simulink model "app_Main10msMgr"  (R2019b)
settings: Solver=FixedStepDiscrete  StartTime=0.0  StopTime=inf  FixedStep=0.01  RelTol=1e-3  EnableMultiTasking=on
PreLoadFcn:
  | try
  |    tapas_types('load');
  | catch
  |   disp('TAPAS WARNING: Tapas Types could not be loaded ...');
  | end
  | 
  | try
  |   app_types('load');
  | catch
  |   currdir =pwd;
  |   try
  |     cd('..\app_types\');
  |     app_types('load');
  |     cd(currdir);
  |   catch
  |     try
  |        cd('..\..\app_types\');
  |        app_types('load');
  |        cd(currdir);
  |     catch
  |        cd(currdir);
  |        disp('TAPAS WARNING: Application Types could not be loaded ...');
  |     end
  |   end
  |   try
  |       clear currdir;
  |   catch
  |      %Do nothing
  |   end
  | end
libraries: Lib_SiftProbe_deVCU_IO x44, Lib_SiftProbe_deVCU_Anlg x23, Lib_SiftProbe_deVCU_Com x4, simulink x4, hdlsllib x1
settings Model: Creator=kmansour  LastModifiedBy=depl_
settings DataIOCC: LimitDataPoints=on  SaveFormat=Array  ReturnWorkspaceOutputs=off
settings OptimizationCC: LifeSpan=1  EfficientTunableParamExpr=on
settings DebuggingCC: AllowSymbolicDim=off  SFUnexpectedBacktrackingDiag=warning  SFNoUnconditionalDefaultTransitionDiag=warning  SFExecutionAtInitializationDiag=none  ArithmeticOperatorsInVariantConditions=warning
settings HardwareCC: ProdBitPerPointer=32  ProdBitPerSizeT=32  ProdBitPerPtrDiffT=32  ProdLargestAtomicInteger=Long  ProdLargestAtomicFloat=Double  ProdEndianess=BigEndian  ProdWordSize=32  ProdHWDeviceType=Texas Instruments->TMS570 Cortex-R4
settings ModelReferenceCC: ModelReferenceNumInstancesAllowed=Single  PropagateSignalLabelsOutOfModel=off
settings SFSimCC: SimUseLocalCustomCode=off  MATLABDynamicMemAlloc=off  CustomCodeUndefinedFunction=UseInterfaceOnly
settings RTWCC: SystemTargetFile=ert.tlc  GenCodeOnly=on  TemplateMakefile=ert_default_tmf  GenerateReport=on  RTWUseLocalCustomCode=off  IncludeHyperlinkInReport=on  LaunchReport=on  GenerateTraceInfo=on  GenerateTraceReport=on  GenerateTraceReportSl=on  GenerateTraceReportSf=on  GenerateTraceReportEml=on  CheckMdlBeforeBuild=Warning
settings CodeAppCC: IgnoreCustomStorageClasses=off  MaxIdLength=63  StateflowObjectComments=on
settings ERTTargetCC: MultiwordLength=2048  GenerateSampleERTMain=on  SuppressErrorStatus=on  GenerateASAP2=on  RTWCAPISignals=on  RTWCAPIParams=on  RTWCAPIStates=on  RTWCAPIRootIO=on  ERTSrcFileBannerTemplate=deMCD_code_template.cgt  ERTHdrFileBannerTemplate=deMCD_code_template.cgt  ERTDataSrcFileTemplate=deMCD_code_template.cgt  ERTDataHdrFileTemplate=deMCD_code_template.cgt  ERTCustomFileTemplate=example_file_process.tlc  ConvertIfToSwitch=off  SuppressUnreachableDefaultCases=off
settings ConfigComp: CovMetricSettings=dw  CovHtmlReporting=on  CovSaveCumulativeToWorkspaceVar=on  CovSaveSingleToWorkspaceVar=on  CovExternalEMLEnable=off

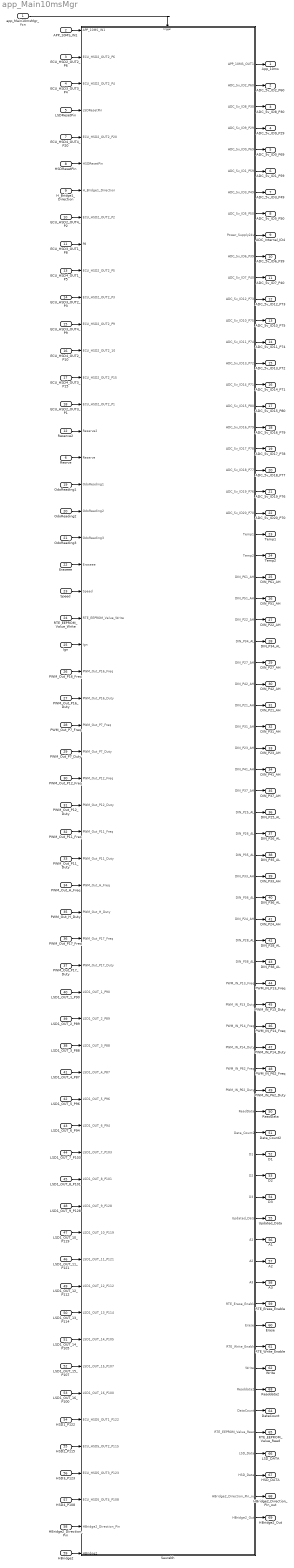
== system app_Main10msMgr ==
  app_Main10msMgr_fcn : Inport  SampleTime=10e-3  OutputFunctionCall=on
  APP_10MS_IN1 : Inport  Port=2
  ECU_HSD2_OUT2_P6 : Inport  Port=3
  ECU_HSD3_OUT3_P4 : Inport  Port=4
  LSDResetPin : Inport  Port=5
  Resrve : Inport  Port=6
  ECU_HSD4_OUT4_P20 : Inport  Port=7
  HSDResetPin : Inport  Port=8
  H_Bridge1_Direction : Inport  Port=9
  ECU_HSD2_OUT4_P2 : Inport  Port=10
  ECU_HSD3_OUT1_P8 : Inport  Port=11
  Reserve2 : Inport  Port=12
  ECU_HSD4_OUT1_P5 : Inport  Port=13
  ECU_HSD3_OUT2_P3 : Inport  Port=14
  ECU_HSD3_OUT4_P9 : Inport  Port=15
  ECU_HSD4_OUT2_P10 : Inport  Port=16
  ECU_HSD4_OUT3_P15 : Inport  Port=17
  ECU_HSD2_OUT3_P1 : Inport  Port=18
  OdoReading1 : Inport  Port=19
  OdoReading2 : Inport  Port=20
  OdoReading3 : Inport  Port=21
  Eraseee : Inport  Port=22
  Speed : Inport  Port=23
  RTE_EEPROM_Value_Write : Inport  Port=24
  Ign : Inport  Port=25
  PWM_Out_P16_Freq : Inport  Port=26
  PWM_Out_P16_Duty : Inport  Port=27
  PWM_Out_P7_Freq : Inport  Port=28
  PWM_Out_P7_Duty : Inport  Port=29
  PWM_Out_P12_Freq : Inport  Port=30
  PWM_Out_P12_Duty : Inport  Port=31
  PWM_Out_P11_Freq : Inport  Port=32
  PWM_Out_P11_Duty : Inport  Port=33
  PWM_Out_H_Freq : Inport  Port=34
  PWM_Out_H_Duty : Inport  Port=35
  PWM_Out_P17_Freq : Inport  Port=36
  PWM_Out_P17_Duty : Inport  Port=37
  LSD1_OUT_3_P88 : Inport  Port=38
  LSD1_OUT_2_P89 : Inport  Port=39
  LSD1_OUT_1_P90 : Inport  Port=40
  LSD1_OUT_4_P87 : Inport  Port=41
  LSD1_OUT_5_P96 : Inport  Port=42
  LSD1_OUT_6_P94 : Inport  Port=43
  LSD1_OUT_7_P103 : Inport  Port=44
  LSD1_OUT_8_P101 : Inport  Port=45
  LSD1_OUT_11_P121 : Inport  Port=46
  LSD1_OUT_10_P119 : Inport  Port=47
  LSD1_OUT_9_P128 : Inport  Port=48
  LSD1_OUT_12_P112 : Inport  Port=49
  LSD1_OUT_13_P114 : Inport  Port=50
  LSD1_OUT_14_P105 : Inport  Port=51
  LSD1_OUT_15_P107 : Inport  Port=52
  LSD1_OUT_16_P100 : Inport  Port=53
  HSD1_P122 : Inport  Port=54
  HSD2_P115 : Inport  Port=55
  HSD3_P123 : Inport  Port=56
  HSD4_P108 : Inport  Port=57
  HBridge2_Direction_Pin : Inport  Port=58
  HBridge2 : Inport  Port=59
  Saurabh : Subsystem
      mask Display: image(('Devise Logo.JPG'),'center');
  App_10ms : Outport
  ADC_5v_ID2_P60 : Outport  Port=2
  ADC_5v_ID8_P30 : Outport  Port=3
  ADC_5v_ID9_P29 : Outport  Port=4
  ADC_5v_ID0_P69 : Outport  Port=5
  ADC_5v_ID1_P59 : Outport  Port=6
  ADC_5v_ID3_P49 : Outport  Port=7
  ADC_5v_ID5_P50 : Outport  Port=8
  ADC_Internal_ID4 : Outport  Port=9
  ADC_5v_ID6_P39 : Outport  Port=10
  ADC_5v_ID7_P40 : Outport  Port=11
  ADC_5v_ID12_P73 : Outport  Port=12
  ADC_5v_ID10_P75 : Outport  Port=13
  ADC_5v_ID11_P74 : Outport  Port=14
  ADC_5v_ID13_P72 : Outport  Port=15
  ADC_5v_ID14_P71 : Outport  Port=16
  ADC_5v_ID15_P80 : Outport  Port=17
  ADC_5v_ID16_P79 : Outport  Port=18
  ADC_5v_ID17_P78 : Outport  Port=19
  ADC_5v_ID18_P77 : Outport  Port=20
  ADC_5v_ID19_P76 : Outport  Port=21
  ADC_5v_ID20_P70 : Outport  Port=22
  Temp1 : Outport  Port=23
  Temp2 : Outport  Port=24
  DIN_P61_AH : Outport  Port=25
  DIN_P51_AH : Outport  Port=26
  DIN_P22_AH : Outport  Port=27
  DIN_P34_AL : Outport  Port=28
  DIN_P27_AH : Outport  Port=29
  DIN_P42_AH : Outport  Port=30
  DIN_P21_AH : Outport  Port=31
  DIN_P31_AH : Outport  Port=32
  DIN_P23_AH : Outport  Port=33
  DIN_P41_AH : Outport  Port=34
  DIN_P37_AH : Outport  Port=35
  DIN_P25_AL : Outport  Port=36
  DIN_P26_AL : Outport  Port=37
  DIN_P35_AL : Outport  Port=38
  DIN_P33_AH : Outport  Port=39
  DIN_P36_AL : Outport  Port=40
  DIN_P24_AH : Outport  Port=41
  DIN_P28_AL : Outport  Port=42
  DIN_P38_AL : Outport  Port=43
  PWM_IN_P13_Freq : Outport  Port=44
  PWM_IN_P13_Duty : Outport  Port=45
  PWM_IN_P14_Freq : Outport  Port=46
  PWM_IN_P14_Duty : Outport  Port=47
  PWM_IN_P62_Freq : Outport  Port=48
  PWM_IN_P62_Duty : Outport  Port=49
  ReadData : Outport  Port=50
  Data_Count2 : Outport  Port=51
  D1 : Outport  Port=52
  D2 : Outport  Port=53
  D3 : Outport  Port=54
  Updated_Data : Outport  Port=55
  A1 : Outport  Port=56
  A2 : Outport  Port=57
  A3 : Outport  Port=58
  RTE_Erase_Enable : Outport  Port=59
  Erase : Outport  Port=60
  RTE_Write_Enable : Outport  Port=61
  Write : Outport  Port=62
  Readdata2 : Outport  Port=63
  DataCount : Outport  Port=64
  RTE_EEPROM_Value_Read : Outport  Port=65
  LSD_DATA : Outport  Port=66
  HSD_DATA : Outport  Port=67
  HBridge2_Direction_Pin_out : Outport  Port=68
  HBridge2_Out : Outport  Port=69
  wires:
  Saurabh/44(PWM_IN_P13_Freq) -> PWM_IN_P13_Freq/1
  Saurabh/67(HSD_Data) -> HSD_DATA/1
  Saurabh/62(Write) -> Write/1
  Saurabh/66(LSD_Data) -> LSD_DATA/1
  LSD1_OUT_13_P114/1 -> Saurabh/49("LSD1_OUT_13_P114 ")
  LSD1_OUT_1_P90/1 -> Saurabh/37(LSD1_OUT_1_P90)
  LSD1_OUT_12_P112/1 -> Saurabh/48("LSD1_OUT_12_P112 ")
  Eraseee/1 -> Saurabh/21(Eraseee)
  Saurabh/53(D2) -> D2/1
  OdoReading1/1 -> Saurabh/18(OdoReading1)
  Saurabh/40(DIN_P36_AL) -> DIN_P36_AL/1
  PWM_Out_P17_Freq/1 -> Saurabh/35(PWM_Out_P17_Freq)
  LSD1_OUT_10_P119/1 -> Saurabh/46("LSD1_OUT_10_P119 ")
  LSD1_OUT_9_P128/1 -> Saurabh/45("LSD1_OUT_9_P128 ")
  LSD1_OUT_8_P101/1 -> Saurabh/44("LSD1_OUT_8_P101 ")
  LSD1_OUT_14_P105/1 -> Saurabh/50("LSD1_OUT_14_P105 ")
  PWM_Out_H_Freq/1 -> Saurabh/33(PWM_Out_H_Freq)
  LSD1_OUT_15_P107/1 -> Saurabh/51("LSD1_OUT_15_P107 ")
  LSD1_OUT_11_P121/1 -> Saurabh/47("LSD1_OUT_11_P121 ")
  Ign/1 -> Saurabh/24(Ign)
  PWM_Out_P11_Freq/1 -> Saurabh/31(PWM_Out_P11_Freq)
  LSD1_OUT_16_P100/1 -> Saurabh/52(LSD1_OUT_16_P100)
  LSD1_OUT_6_P94/1 -> Saurabh/42("LSD1_OUT_6_P94 ")
  PWM_Out_P16_Freq/1 -> Saurabh/25(PWM_Out_P16_Freq)
  LSD1_OUT_2_P89/1 -> Saurabh/38(LSD1_OUT_2_P89)
  PWM_Out_P7_Duty/1 -> Saurabh/28(PWM_Out_P7_Duty)
  LSD1_OUT_4_P87/1 -> Saurabh/40("LSD1_OUT_4_P87 ")
  LSD1_OUT_5_P96/1 -> Saurabh/41("LSD1_OUT_5_P96 ")
  LSD1_OUT_7_P103/1 -> Saurabh/43("LSD1_OUT_7_P103 ")
  LSD1_OUT_3_P88/1 -> Saurabh/39("LSD1_OUT_3_P88 ")
  PWM_Out_P12_Freq/1 -> Saurabh/29(PWM_Out_P12_Freq)
  PWM_Out_P16_Duty/1 -> Saurabh/26(PWM_Out_P16_Duty)
  PWM_Out_P7_Freq/1 -> Saurabh/27(PWM_Out_P7_Freq)
  PWM_Out_P17_Duty/1 -> Saurabh/36(PWM_Out_P17_Duty)
  PWM_Out_H_Duty/1 -> Saurabh/34(PWM_Out_H_Duty)
  PWM_Out_P11_Duty/1 -> Saurabh/32(PWM_Out_P11_Duty)
  PWM_Out_P12_Duty/1 -> Saurabh/30(PWM_Out_P12_Duty)
  Saurabh/65(RTE_EEPROM_Value_Read) -> RTE_EEPROM_Value_Read/1
  Saurabh/64(DataCount) -> DataCount/1
  Speed/1 -> Saurabh/22(Speed)
  Saurabh/63(Readdata2) -> Readdata2/1
  Saurabh/61(RTE_Write_Enable) -> RTE_Write_Enable/1
  RTE_EEPROM_Value_Write/1 -> Saurabh/23(RTE_EEPROM_Value_Write)
  ECU_HSD4_OUT4_P20/1 -> Saurabh/5(ECU_HSD2_OUT2_P20)
  Saurabh/60(Erase) -> Erase/1
  Saurabh/59(RTE_Erase_Enable) -> RTE_Erase_Enable/1
  Saurabh/55(Updated_Data) -> Updated_Data/1
  Saurabh/58(A3) -> A3/1
  Saurabh/48(PWM_IN_P62_Freq) -> PWM_IN_P62_Freq/1
  Saurabh/57(A2) -> A2/1
  Saurabh/56(A1) -> A1/1
  Saurabh/52(D1) -> D1/1
  Saurabh/54(D3) -> D3/1
  Saurabh/46(PWM_IN_P14_Freq) -> PWM_IN_P14_Freq/1
  Saurabh/51(Data_Count2) -> Data_Count2/1
  Saurabh/50(ReadData) -> ReadData/1
  OdoReading2/1 -> Saurabh/19(OdoReading2)
  OdoReading3/1 -> Saurabh/20(OdoReading3)
  Saurabh/47(PWM_IN_P14_Duty) -> PWM_IN_P14_Duty/1
  Saurabh/49(PWM_IN_P62_Duty) -> PWM_IN_P62_Duty/1
  Saurabh/45(PWM_IN_P13_Duty) -> PWM_IN_P13_Duty/1
  Saurabh/36(DIN_P25_AL) -> DIN_P25_AL/1
  Saurabh/39(DIN_P33_AH) -> DIN_P33_AH/1
  Saurabh/42(DIN_P28_AL) -> DIN_P28_AL/1
  Saurabh/38(DIN_P35_AL) -> DIN_P35_AL/1
  Saurabh/37(DIN_P26_AL) -> DIN_P26_AL/1
  Saurabh/41(DIN_P24_AH) -> DIN_P24_AH/1
  Saurabh/35(DIN_P37_AH) -> DIN_P37_AH/1
  Saurabh/43(DIN_P38_AL) -> DIN_P38_AL/1
  Saurabh/29(DIN_P27_AH) -> DIN_P27_AH/1
  Saurabh/25(DIN_P61_AH) -> DIN_P61_AH/1
  Saurabh/31(DIN_P21_AH) -> DIN_P21_AH/1
  Saurabh/34(DIN_P41_AH) -> DIN_P41_AH/1
  Saurabh/32(DIN_P31_AH) -> DIN_P31_AH/1
  Saurabh/26(DIN_P51_AH) -> DIN_P51_AH/1
  Saurabh/30(DIN_P42_AH) -> DIN_P42_AH/1
  Saurabh/27(DIN_P22_AH) -> DIN_P22_AH/1
  Saurabh/28(DIN_P34_AL) -> DIN_P34_AL/1
  Saurabh/33(DIN_P23_AH) -> DIN_P23_AH/1
  ECU_HSD2_OUT3_P1/1 -> Saurabh/15(ECU_HSD2_OUT2_P1)
  ECU_HSD4_OUT2_P10/1 -> Saurabh/13(ECU_HSD2_OUT2_10)
  ECU_HSD4_OUT1_P5/1 -> Saurabh/10(ECU_HSD2_OUT2_P5)
  ECU_HSD3_OUT4_P9/1 -> Saurabh/12(ECU_HSD2_OUT2_P9)
  ECU_HSD3_OUT2_P3/1 -> Saurabh/11(ECU_HSD2_OUT2_P3)
  ECU_HSD4_OUT3_P15/1 -> Saurabh/14(ECU_HSD2_OUT2_P15)
  Reserve2/1 -> Saurabh/16(Reserve2)
  ECU_HSD3_OUT1_P8/1 -> Saurabh/9(P8)
  ECU_HSD2_OUT4_P2/1 -> Saurabh/8(ECU_HSD2_OUT2_P2)
  H_Bridge1_Direction/1 -> Saurabh/7(H_Bridge1_Direction)
  HSDResetPin/1 -> Saurabh/6(HSDResetPin)
  Resrve/1 -> Saurabh/17(Reserve)
  LSDResetPin/1 -> Saurabh/4(LSDResetPin)
  ECU_HSD3_OUT3_P4/1 -> Saurabh/3(ECU_HSD2_OUT2_P4)
  ECU_HSD2_OUT2_P6/1 -> Saurabh/2(ECU_HSD2_OUT2_P6)
  Saurabh/24(Temp2) -> Temp2/1
  Saurabh/23(Temp1) -> Temp1/1
  Saurabh/15(ADC_5v_ID13_P72) -> ADC_5v_ID13_P72/1
  Saurabh/18(ADC_5v_ID16_P79) -> ADC_5v_ID16_P79/1
  Saurabh/14(ADC_5v_ID11_P74) -> ADC_5v_ID11_P74/1
  Saurabh/16(ADC_5v_ID14_P71) -> ADC_5v_ID14_P71/1
  Saurabh/22(ADC_5v_ID20_P70) -> ADC_5v_ID20_P70/1
  Saurabh/21(ADC_5v_ID19_P76) -> ADC_5v_ID19_P76/1
  Saurabh/20(ADC_5v_ID18_P77) -> ADC_5v_ID18_P77/1
  Saurabh/17(ADC_5v_ID15_P80) -> ADC_5v_ID15_P80/1
  Saurabh/19(ADC_5v_ID17_P78) -> ADC_5v_ID17_P78/1
  Saurabh/12(ADC_5v_ID12_P73) -> ADC_5v_ID12_P73/1
  Saurabh/10(ADC_5v_ID6_P39) -> ADC_5v_ID6_P39/1
  Saurabh/6(ADC_5v_ID1_P59) -> ADC_5v_ID1_P59/1
  Saurabh/13(ADC_5v_ID10_P75) -> ADC_5v_ID10_P75/1
  Saurabh/9(Power_Supply24v) -> ADC_Internal_ID4/1
  Saurabh/2(ADC_5v_ID2_P60) -> ADC_5v_ID2_P60/1
  Saurabh/11(ADC_5v_ID7_P40) -> ADC_5v_ID7_P40/1
  Saurabh/7(ADC_5v_ID3_P49) -> ADC_5v_ID3_P49/1
  Saurabh/8(ADC_5v_ID5_P50) -> ADC_5v_ID5_P50/1
  Saurabh/4(ADC_5v_ID9_P29) -> ADC_5v_ID9_P29/1
  Saurabh/3(ADC_5v_ID8_P30) -> ADC_5v_ID8_P30/1
  Saurabh/5(ADC_5v_ID0_P69) -> ADC_5v_ID0_P69/1
  Saurabh/1(APP_10MS_OUT1) -> App_10ms/1
  APP_10MS_IN1/1 -> Saurabh/1(APP_10MS_IN1)
  app_Main10msMgr_fcn/1 -> Saurabh/Trigger
  HSD1_P122/1 -> Saurabh/53(ECU_HSD5_OUT1_P122)
  HSD2_P115/1 -> Saurabh/54(ECU_HSD5_OUT2_P115)
  HSD3_P123/1 -> Saurabh/55("ECU_HSD5_OUT3_P123 ")
  HSD4_P108/1 -> Saurabh/56(ECU_HSD5_OUT4_P108)
  HBridge2_Direction_Pin/1 -> Saurabh/57(HBridge2_Direction_Pin)
  HBridge2/1 -> Saurabh/58(HBridge2)
  Saurabh/68(HBridge2_Direction_Pin_out) -> HBridge2_Direction_Pin_out/1
  Saurabh/69(HBridge2_Out) -> HBridge2_Out/1

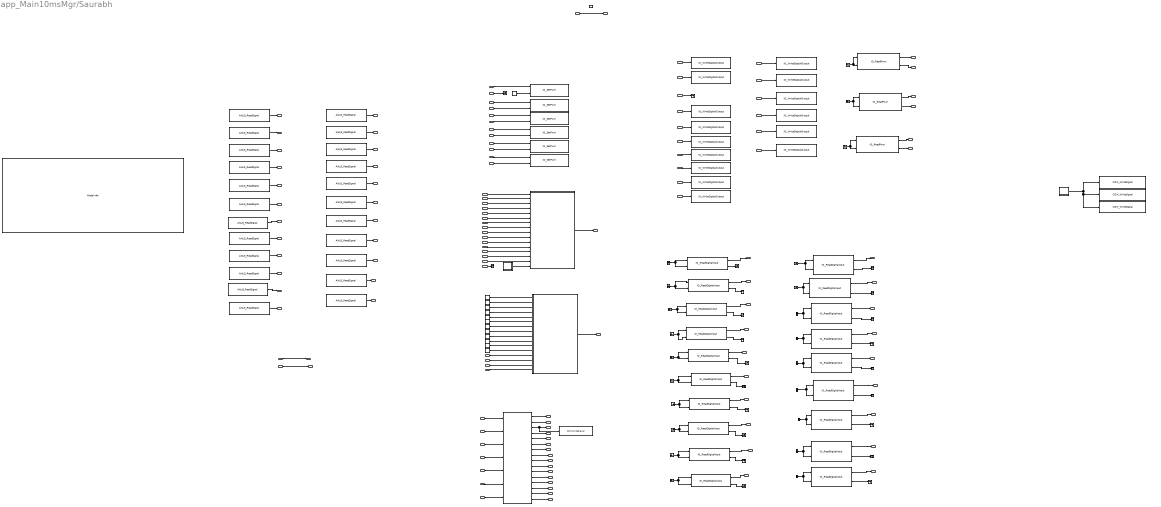
== system app_Main10msMgr/Saurabh ==
  note: CAN_Channel
  note: H_bridge2
  note: HSD
  note: LSD
  note: PWM_IN
  note: EPROM
  note: DigitalInputs
  note: DigitalOutput
  note: PWMOut
  note: ADC
  note: (C) 2020-2021 Devise Electronics Pvt Ltd
      | All rights reserved.
      |
      | All data and information contained in or disclosed by this document is confidential and proprietary information of Devise Electronics Pvt Ltd and all rights therein are expressly reserved. By accepting this material the recipient agrees that this material and the information contained therein is held in confidence and in trust and will not be used, copied, reproduced in whole or in part, nor its contents revealed in any manner to others without the express written permission of Devise Electronics Pvt Ltd
      |
      | Author:
      |
      | Devise Electronics Pvt Ltd
      | Pune,
      | India
      | E-mail: Shekhar.malani@deviseelectronics.com
  APP_10MS_IN1 : Inport
  ECU_HSD2_OUT2_P6 : Inport  Port=2
  ECU_HSD2_OUT2_P4 : Inport  Port=3
  LSDResetPin : Inport  Port=4
  ECU_HSD2_OUT2_P20 : Inport  Port=5
  HSDResetPin : Inport  Port=6
  H_Bridge1_Direction : Inport  Port=7
  ECU_HSD2_OUT2_P2 : Inport  Port=8
  P8 : Inport  Port=9
  ECU_HSD2_OUT2_P5 : Inport  Port=10
  ECU_HSD2_OUT2_P3 : Inport  Port=11
  ECU_HSD2_OUT2_P9 : Inport  Port=12
  ECU_HSD2_OUT2_10 : Inport  Port=13
  ECU_HSD2_OUT2_P15 : Inport  Port=14
  ECU_HSD2_OUT2_P1 : Inport  Port=15
  Reserve2 : Inport  Port=16
  Reserve : Inport  Port=17
  OdoReading1 : Inport  Port=18
  OdoReading2 : Inport  Port=19
  OdoReading3 : Inport  Port=20
  Eraseee : Inport  Port=21
  Speed : Inport  Port=22
  RTE_EEPROM_Value_Write : Inport  Port=23
  Ign : Inport  Port=24
  PWM_Out_P16_Freq : Inport  Port=25
  PWM_Out_P16_Duty : Inport  Port=26
  PWM_Out_P7_Freq : Inport  Port=27
  PWM_Out_P7_Duty : Inport  Port=28
  PWM_Out_P12_Freq : Inport  Port=29
  PWM_Out_P12_Duty : Inport  Port=30
  PWM_Out_P11_Freq : Inport  Port=31
  PWM_Out_P11_Duty : Inport  Port=32
  PWM_Out_H_Freq : Inport  Port=33
  PWM_Out_H_Duty : Inport  Port=34
  PWM_Out_P17_Freq : Inport  Port=35
  PWM_Out_P17_Duty : Inport  Port=36
  LSD1_OUT_1_P90 : Inport  Port=37
  LSD1_OUT_2_P89 : Inport  Port=38
  "LSD1_OUT_3_P88 " : Inport  Port=39
  "LSD1_OUT_4_P87 " : Inport  Port=40
  "LSD1_OUT_5_P96 " : Inport  Port=41
  "LSD1_OUT_6_P94 " : Inport  Port=42
  "LSD1_OUT_7_P103 " : Inport  Port=43
  "LSD1_OUT_8_P101 " : Inport  Port=44
  "LSD1_OUT_9_P128 " : Inport  Port=45
  "LSD1_OUT_10_P119 " : Inport  Port=46
  "LSD1_OUT_11_P121 " : Inport  Port=47
  "LSD1_OUT_12_P112 " : Inport  Port=48
  "LSD1_OUT_13_P114 " : Inport  Port=49
  "LSD1_OUT_14_P105 " : Inport  Port=50
  "LSD1_OUT_15_P107 " : Inport  Port=51
  LSD1_OUT_16_P100 : Inport  Port=52
  ECU_HSD5_OUT1_P122 : Inport  Port=53
  ECU_HSD5_OUT2_P115 : Inport  Port=54
  "ECU_HSD5_OUT3_P123 " : Inport  Port=55
  ECU_HSD5_OUT4_P108 : Inport  Port=56
  HBridge2_Direction_Pin : Inport  Port=57
  HBridge2 : Inport  Port=58
  Trigger : TriggerPort  TriggerType=function-call  VariantControl=Variant  SampleTimeType=periodic  SampleTime=-1  PortDimensions=1
  ANLG_ReadSignal : Lib_SiftProbe_deVCU_Anlg/ANLG_ReadSignal  PARAM_ID=ECU_ANLG_ADC_5V_P60
      settings: SourceProductName=deMCD - SiftProbe_deVCU
  ANLG_ReadSignal1 : Lib_SiftProbe_deVCU_Anlg/ANLG_ReadSignal  PARAM_ID=ECU_ANLG_ADC_5V_P30
      settings: SourceProductName=deMCD - SiftProbe_deVCU
  ANLG_ReadSignal10 : Lib_SiftProbe_deVCU_Anlg/ANLG_ReadSignal  PARAM_ID=ECU_ANLG_ADC_5V_P73
      settings: SourceProductName=deMCD - SiftProbe_deVCU
  ANLG_ReadSignal11 : Lib_SiftProbe_deVCU_Anlg/ANLG_ReadSignal  PARAM_ID=ECU_ANLG_ADC_5V_P75
      settings: SourceProductName=deMCD - SiftProbe_deVCU
  ANLG_ReadSignal12 : Lib_SiftProbe_deVCU_Anlg/ANLG_ReadSignal  PARAM_ID=ECU_ANLG_ADC_5V_P74
      settings: SourceProductName=deMCD - SiftProbe_deVCU
  ANLG_ReadSignal13 : Lib_SiftProbe_deVCU_Anlg/ANLG_ReadSignal  PARAM_ID=ECU_ANLG_ADC_5V_P72
      settings: SourceProductName=deMCD - SiftProbe_deVCU
  ANLG_ReadSignal14 : Lib_SiftProbe_deVCU_Anlg/ANLG_ReadSignal  PARAM_ID=ECU_ANLG_ADC_5V_P71
      settings: SourceProductName=deMCD - SiftProbe_deVCU
  ANLG_ReadSignal15 : Lib_SiftProbe_deVCU_Anlg/ANLG_ReadSignal  PARAM_ID=ECU_ANLG_ADC_5V_P80
      settings: SourceProductName=deMCD - SiftProbe_deVCU
  ANLG_ReadSignal16 : Lib_SiftProbe_deVCU_Anlg/ANLG_ReadSignal  PARAM_ID=ECU_ANLG_ADC_5V_P79
      settings: SourceProductName=deMCD - SiftProbe_deVCU
  ANLG_ReadSignal17 : Lib_SiftProbe_deVCU_Anlg/ANLG_ReadSignal  PARAM_ID=ECU_ANLG_ADC_5V_P78
      settings: SourceProductName=deMCD - SiftProbe_deVCU
  ANLG_ReadSignal18 : Lib_SiftProbe_deVCU_Anlg/ANLG_ReadSignal  PARAM_ID=ECU_ANLG_ADC_5V_P77
      settings: SourceProductName=deMCD - SiftProbe_deVCU
  ANLG_ReadSignal19 : Lib_SiftProbe_deVCU_Anlg/ANLG_ReadSignal  PARAM_ID=ECU_ANLG_ADC_5V_P76
      settings: SourceProductName=deMCD - SiftProbe_deVCU
  ANLG_ReadSignal2 : Lib_SiftProbe_deVCU_Anlg/ANLG_ReadSignal  PARAM_ID=ECU_ANLG_ADC_5V_P29
      settings: SourceProductName=deMCD - SiftProbe_deVCU
  ANLG_ReadSignal20 : Lib_SiftProbe_deVCU_Anlg/ANLG_ReadSignal  PARAM_ID=ECU_ANLG_ADC_5V_P70
      settings: SourceProductName=deMCD - SiftProbe_deVCU
  ANLG_ReadSignal21 : Lib_SiftProbe_deVCU_Anlg/ANLG_ReadSignal  PARAM_ID=ECU_ANLG_TEMP_SENSOR1
      settings: SourceProductName=deMCD - SiftProbe_deVCU
  ANLG_ReadSignal22 : Lib_SiftProbe_deVCU_Anlg/ANLG_ReadSignal  PARAM_ID=ECU_ANLG_TEMP_SENSOR2
      settings: SourceProductName=deMCD - SiftProbe_deVCU
  ANLG_ReadSignal3 : Lib_SiftProbe_deVCU_Anlg/ANLG_ReadSignal  PARAM_ID=ECU_ANLG_ADC_5V_P69
      settings: SourceProductName=deMCD - SiftProbe_deVCU
  ANLG_ReadSignal4 : Lib_SiftProbe_deVCU_Anlg/ANLG_ReadSignal  PARAM_ID=ECU_ANLG_ADC_5V_P59
      settings: SourceProductName=deMCD - SiftProbe_deVCU
  ANLG_ReadSignal5 : Lib_SiftProbe_deVCU_Anlg/ANLG_ReadSignal  PARAM_ID=ECU_ANLG_ADC_5V_P49
      settings: SourceProductName=deMCD - SiftProbe_deVCU
  ANLG_ReadSignal6 : Lib_SiftProbe_deVCU_Anlg/ANLG_ReadSignal  PARAM_ID=ECU_ANLG_ADC_5V_P50
      settings: SourceProductName=deMCD - SiftProbe_deVCU
  ANLG_ReadSignal7 : Lib_SiftProbe_deVCU_Anlg/ANLG_ReadSignal  PARAM_ID=ECU_ANLG_POWER_SUPPLY24V
      settings: SourceProductName=deMCD - SiftProbe_deVCU
  ANLG_ReadSignal8 : Lib_SiftProbe_deVCU_Anlg/ANLG_ReadSignal  PARAM_ID=ECU_ANLG_ADC_5V_P39
      settings: SourceProductName=deMCD - SiftProbe_deVCU
  ANLG_ReadSignal9 : Lib_SiftProbe_deVCU_Anlg/ANLG_ReadSignal  PARAM_ID=ECU_ANLG_ADC_5V_P40
      settings: SourceProductName=deMCD - SiftProbe_deVCU
  COM_WriteSignal49 : Lib_SiftProbe_deVCU_Com/COM_WriteSignal  PARAM_ID=APP_TX_CAN2_SIGNAL
      settings: SourceProductName=deMCD - SiftProbe_deVCU
  COM_WriteSignal50 : Lib_SiftProbe_deVCU_Com/COM_WriteSignal  PARAM_ID=APP_TX_CAN3_SIGNAL
      settings: SourceProductName=deMCD - SiftProbe_deVCU
  COM_WriteSignal52 : Lib_SiftProbe_deVCU_Com/COM_WriteSignal  PARAM_ID=APP_TX_CAN1_SIGNAL
      settings: SourceProductName=deMCD - SiftProbe_deVCU
  COM_WriteSignal53 : Lib_SiftProbe_deVCU_Com/COM_WriteSignal  PARAM_ID=APP_TX_ADC_P29
      settings: SourceProductName=deMCD - SiftProbe_deVCU
  Chart : Stateflow chart  BlockKeywords=__PRM__SERIALIZED__DATA__:Stateflow Chart,Stateflow Diagram  TreatAsAtomicUnit=on
  Chart1 : Stateflow chart  BlockKeywords=__PRM__SERIALIZED__DATA__:Stateflow Chart,Stateflow Diagram  TreatAsAtomicUnit=on
  Constant : Constant
  Constant1 : Constant
  Constant{3..11} (9 alike) : Constant  Value=0
  Constant12 : Constant  Value=50
  Constant2 : Constant
  Ground{,1..21} (22 alike) : Ground
  HSD : Subsystem
  IO_ReadDigitalInput : Lib_SiftProbe_deVCU_IO/IO_ReadDigitalInput  PARAM_ID=ECU_DIN_AUX_61_H_DI
      settings: SourceProductName=deMCD - SiftProbe_deVCU
  IO_ReadDigitalInput1 : Lib_SiftProbe_deVCU_IO/IO_ReadDigitalInput  PARAM_ID=ECU_DIN_AUX_51_H_DI
      settings: SourceProductName=deMCD - SiftProbe_deVCU
  IO_ReadDigitalInput10 : Lib_SiftProbe_deVCU_IO/IO_ReadDigitalInput  PARAM_ID=ECU_DIN_AUX_26_L_DI
      settings: SourceProductName=deMCD - SiftProbe_deVCU
  IO_ReadDigitalInput11 : Lib_SiftProbe_deVCU_IO/IO_ReadDigitalInput  PARAM_ID=ECU_DIN_AUX_35_L_DI
      settings: SourceProductName=deMCD - SiftProbe_deVCU
  IO_ReadDigitalInput12 : Lib_SiftProbe_deVCU_IO/IO_ReadDigitalInput  PARAM_ID=ECU_DIN_AUX_33_H_DI
      settings: SourceProductName=deMCD - SiftProbe_deVCU
  IO_ReadDigitalInput13 : Lib_SiftProbe_deVCU_IO/IO_ReadDigitalInput  PARAM_ID=ECU_DIN_AUX_36_L_DI
      settings: SourceProductName=deMCD - SiftProbe_deVCU
  IO_ReadDigitalInput14 : Lib_SiftProbe_deVCU_IO/IO_ReadDigitalInput  PARAM_ID=ECU_DIN_AUX_24_H_DI
      settings: SourceProductName=deMCD - SiftProbe_deVCU
  IO_ReadDigitalInput15 : Lib_SiftProbe_deVCU_IO/IO_ReadDigitalInput  PARAM_ID=ECU_DIN_AUX_23_H_DI
      settings: SourceProductName=deMCD - SiftProbe_deVCU
  IO_ReadDigitalInput16 : Lib_SiftProbe_deVCU_IO/IO_ReadDigitalInput  PARAM_ID=ECU_DIN_AUX_28_L_DI
      settings: SourceProductName=deMCD - SiftProbe_deVCU
  IO_ReadDigitalInput17 : Lib_SiftProbe_deVCU_IO/IO_ReadDigitalInput  PARAM_ID=ECU_DIN_AUX_41_H_DI
      settings: SourceProductName=deMCD - SiftProbe_deVCU
  IO_ReadDigitalInput18 : Lib_SiftProbe_deVCU_IO/IO_ReadDigitalInput  PARAM_ID=ECU_DIN_AUX_38_L_DI
      settings: SourceProductName=deMCD - SiftProbe_deVCU
  IO_ReadDigitalInput2 : Lib_SiftProbe_deVCU_IO/IO_ReadDigitalInput  PARAM_ID=ECU_DIN_AUX_22_H_DI
      settings: SourceProductName=deMCD - SiftProbe_deVCU
  IO_ReadDigitalInput3 : Lib_SiftProbe_deVCU_IO/IO_ReadDigitalInput  PARAM_ID=ECU_DIN_AUX_34_L_DI
      settings: SourceProductName=deMCD - SiftProbe_deVCU
  IO_ReadDigitalInput4 : Lib_SiftProbe_deVCU_IO/IO_ReadDigitalInput  PARAM_ID=ECU_DIN_AUX_27_H_DI
      settings: SourceProductName=deMCD - SiftProbe_deVCU
  IO_ReadDigitalInput5 : Lib_SiftProbe_deVCU_IO/IO_ReadDigitalInput  PARAM_ID=ECU_DIN_AUX_42_H_DI
      settings: SourceProductName=deMCD - SiftProbe_deVCU
  IO_ReadDigitalInput6 : Lib_SiftProbe_deVCU_IO/IO_ReadDigitalInput  PARAM_ID=ECU_DIN_AUX_21_H_DI
      settings: SourceProductName=deMCD - SiftProbe_deVCU
  IO_ReadDigitalInput7 : Lib_SiftProbe_deVCU_IO/IO_ReadDigitalInput  PARAM_ID=ECU_DIN_AUX_31_H_DI
      settings: SourceProductName=deMCD - SiftProbe_deVCU
  IO_ReadDigitalInput8 : Lib_SiftProbe_deVCU_IO/IO_ReadDigitalInput  PARAM_ID=ECU_DIN_AUX_37_H_DI
      settings: SourceProductName=deMCD - SiftProbe_deVCU
  IO_ReadDigitalInput9 : Lib_SiftProbe_deVCU_IO/IO_ReadDigitalInput  PARAM_ID=ECU_DIN_AUX_25_L_DI
      settings: SourceProductName=deMCD - SiftProbe_deVCU
  IO_ReadPwm : Lib_SiftProbe_deVCU_IO/IO_ReadPwm  PARAM_ID=ECU_PIN_NONAME_PIN_P13
      settings: SourceProductName=deMCD - SiftProbe_deVCU
  IO_ReadPwm1 : Lib_SiftProbe_deVCU_IO/IO_ReadPwm  PARAM_ID=ECU_PIN_NONAME_PIN_P14
      settings: SourceProductName=deMCD - SiftProbe_deVCU
  IO_ReadPwm2 : Lib_SiftProbe_deVCU_IO/IO_ReadPwm  PARAM_ID=ECU_PIN_NONAME_PIN_P62
      settings: SourceProductName=deMCD - SiftProbe_deVCU
  IO_SetPwm1 : Lib_SiftProbe_deVCU_IO/IO_SetPwm  PARAM_ID=ECU_POUT_PWM_POUT_P12
      settings: SourceProductName=deMCD - SiftProbe_deVCU
  IO_SetPwm2 : Lib_SiftProbe_deVCU_IO/IO_SetPwm  PARAM_ID=ECU_POUT_PWM_POUT_P11
      settings: SourceProductName=deMCD - SiftProbe_deVCU
  IO_SetPwm3 : Lib_SiftProbe_deVCU_IO/IO_SetPwm  PARAM_ID=ECU_POUT_PWM_POUT_H
      settings: SourceProductName=deMCD - SiftProbe_deVCU
  IO_SetPwm4 : Lib_SiftProbe_deVCU_IO/IO_SetPwm  PARAM_ID=ECU_POUT_PWM_POUT_P17
      settings: SourceProductName=deMCD - SiftProbe_deVCU
  IO_SetPwm5 : Lib_SiftProbe_deVCU_IO/IO_SetPwm  PARAM_ID=ECU_POUT_PWM_POUT_P16
      settings: SourceProductName=deMCD - SiftProbe_deVCU
  IO_SetPwm6 : Lib_SiftProbe_deVCU_IO/IO_SetPwm  PARAM_ID=ECU_POUT_PWM_POUT_P7
      settings: SourceProductName=deMCD - SiftProbe_deVCU
  IO_WriteDigitalOutput1 : Lib_SiftProbe_deVCU_IO/IO_WriteDigitalOutput  PARAM_ID=ECU_DOUT_ECU_HSD3_OUT3_P4
      settings: SourceProductName=deMCD - SiftProbe_deVCU
  IO_WriteDigitalOutput10 : Lib_SiftProbe_deVCU_IO/IO_WriteDigitalOutput  PARAM_ID=ECU_DOUT_ECU_HSD4_OUT1_P5
      settings: SourceProductName=deMCD - SiftProbe_deVCU
  IO_WriteDigitalOutput11 : Lib_SiftProbe_deVCU_IO/IO_WriteDigitalOutput  PARAM_ID=ECU_DOUT_ECU_HSD3_OUT2_P3
      settings: SourceProductName=deMCD - SiftProbe_deVCU
  IO_WriteDigitalOutput12 : Lib_SiftProbe_deVCU_IO/IO_WriteDigitalOutput  PARAM_ID=ECU_DOUT_ECU_HSD3_OUT4_P9
      settings: SourceProductName=deMCD - SiftProbe_deVCU
  IO_WriteDigitalOutput13 : Lib_SiftProbe_deVCU_IO/IO_WriteDigitalOutput  PARAM_ID=ECU_DOUT_ECU_HSD4_OUT2_P10
      settings: SourceProductName=deMCD - SiftProbe_deVCU
  IO_WriteDigitalOutput14 : Lib_SiftProbe_deVCU_IO/IO_WriteDigitalOutput  PARAM_ID=ECU_DOUT_ECU_HSD4_OUT3_P15
      settings: SourceProductName=deMCD - SiftProbe_deVCU
  IO_WriteDigitalOutput15 : Lib_SiftProbe_deVCU_IO/IO_WriteDigitalOutput  PARAM_ID=ECU_DOUT_ECU_HSD2_OUT3_P1
      settings: SourceProductName=deMCD - SiftProbe_deVCU
  IO_WriteDigitalOutput16 : Lib_SiftProbe_deVCU_IO/IO_WriteDigitalOutput  PARAM_ID=ECU_DOUT_ECU_HSD2_OUT2_P6
      settings: SourceProductName=deMCD - SiftProbe_deVCU
  IO_WriteDigitalOutput3 : Lib_SiftProbe_deVCU_IO/IO_WriteDigitalOutput  PARAM_ID=ECU_DOUT_NONAME_PIN_RESERVE1_
      settings: SourceProductName=deMCD - SiftProbe_deVCU
  IO_WriteDigitalOutput4 : Lib_SiftProbe_deVCU_IO/IO_WriteDigitalOutput  PARAM_ID=ECU_DOUT_NONAME_PIN_RESERVE2_
      settings: SourceProductName=deMCD - SiftProbe_deVCU
  IO_WriteDigitalOutput5 : Lib_SiftProbe_deVCU_IO/IO_WriteDigitalOutput  PARAM_ID=ECU_DOUT_ECU_HSD4_OUT4_P20
      settings: SourceProductName=deMCD - SiftProbe_deVCU
  IO_WriteDigitalOutput6 : Lib_SiftProbe_deVCU_IO/IO_WriteDigitalOutput  PARAM_ID=ECU_DOUT_HSD_RESET_PIN
      settings: SourceProductName=deMCD - SiftProbe_deVCU
  IO_WriteDigitalOutput7 : Lib_SiftProbe_deVCU_IO/IO_WriteDigitalOutput  PARAM_ID=ECU_DOUT_H_BRIDGE1_DIRECTION
      settings: SourceProductName=deMCD - SiftProbe_deVCU
  IO_WriteDigitalOutput8 : Lib_SiftProbe_deVCU_IO/IO_WriteDigitalOutput  PARAM_ID=ECU_DOUT_ECU_HSD2_OUT4_P2
      settings: SourceProductName=deMCD - SiftProbe_deVCU
  IO_WriteDigitalOutput9 : Lib_SiftProbe_deVCU_IO/IO_WriteDigitalOutput  PARAM_ID=ECU_DOUT_ECU_HSD3_OUT1_P8
      settings: SourceProductName=deMCD - SiftProbe_deVCU
  LSD : Subsystem
  Model Info : simulink/Model-Wide Utilities/Model Info  Frame=on  DisplayStringWithTags=|  HorizontalTextAlignment=Left  LeftAlignmentValue=0.02
      | File Name: app_Main10msMgr.slx
      |   Description: 
      |   Author: Saurabh kulkarni
      | 
      |   Modified date/ Time: %<ModifiedDate>
      |   Last Modified date/ Time: %<LastModificationDate>
  Subsystem1 : Subsystem
  Terminator{,1..21} (22 alike) : Terminator
  APP_10MS_OUT1 : Outport
  ADC_5v_ID2_P60 : Outport  Port=2
  ADC_5v_ID8_P30 : Outport  Port=3
  ADC_5v_ID9_P29 : Outport  Port=4
  ADC_5v_ID0_P69 : Outport  Port=5
  ADC_5v_ID1_P59 : Outport  Port=6
  ADC_5v_ID3_P49 : Outport  Port=7
  ADC_5v_ID5_P50 : Outport  Port=8
  Power_Supply24v : Outport  Port=9
  ADC_5v_ID6_P39 : Outport  Port=10
  ADC_5v_ID7_P40 : Outport  Port=11
  ADC_5v_ID12_P73 : Outport  Port=12
  ADC_5v_ID10_P75 : Outport  Port=13
  ADC_5v_ID11_P74 : Outport  Port=14
  ADC_5v_ID13_P72 : Outport  Port=15
  ADC_5v_ID14_P71 : Outport  Port=16
  ADC_5v_ID15_P80 : Outport  Port=17
  ADC_5v_ID16_P79 : Outport  Port=18
  ADC_5v_ID17_P78 : Outport  Port=19
  ADC_5v_ID18_P77 : Outport  Port=20
  ADC_5v_ID19_P76 : Outport  Port=21
  ADC_5v_ID20_P70 : Outport  Port=22
  Temp1 : Outport  Port=23
  Temp2 : Outport  Port=24
  DIN_P61_AH : Outport  Port=25
  DIN_P51_AH : Outport  Port=26
  DIN_P22_AH : Outport  Port=27
  DIN_P34_AL : Outport  Port=28
  DIN_P27_AH : Outport  Port=29
  DIN_P42_AH : Outport  Port=30
  DIN_P21_AH : Outport  Port=31
  DIN_P31_AH : Outport  Port=32
  DIN_P23_AH : Outport  Port=33
  DIN_P41_AH : Outport  Port=34
  DIN_P37_AH : Outport  Port=35
  DIN_P25_AL : Outport  Port=36
  DIN_P26_AL : Outport  Port=37
  DIN_P35_AL : Outport  Port=38
  DIN_P33_AH : Outport  Port=39
  DIN_P36_AL : Outport  Port=40
  DIN_P24_AH : Outport  Port=41
  DIN_P28_AL : Outport  Port=42
  DIN_P38_AL : Outport  Port=43
  PWM_IN_P13_Freq : Outport  Port=44
  PWM_IN_P13_Duty : Outport  Port=45
  PWM_IN_P14_Freq : Outport  Port=46
  PWM_IN_P14_Duty : Outport  Port=47
  PWM_IN_P62_Freq : Outport  Port=48
  PWM_IN_P62_Duty : Outport  Port=49
  ReadData : Outport  Port=50
  Data_Count2 : Outport  Port=51
  D1 : Outport  Port=52
  D2 : Outport  Port=53
  D3 : Outport  Port=54
  Updated_Data : Outport  Port=55
  A1 : Outport  Port=56
  A2 : Outport  Port=57
  A3 : Outport  Port=58
  RTE_Erase_Enable : Outport  Port=59
  Erase : Outport  Port=60
  RTE_Write_Enable : Outport  Port=61
  Write : Outport  Port=62
  Readdata2 : Outport  Port=63
  DataCount : Outport  Port=64
  RTE_EEPROM_Value_Read : Outport  Port=65
  LSD_Data : Outport  Port=66
  HSD_Data : Outport  Port=67
  HBridge2_Direction_Pin_out : Outport  Port=68
  HBridge2_Out : Outport  Port=69
  wires:
  APP_10MS_IN1/1 -> APP_10MS_OUT1/1
  ? -> ?
  ANLG_ReadSignal/1 -> ADC_5v_ID2_P60/1
  ANLG_ReadSignal1/1 -> ADC_5v_ID8_P30/1
  ANLG_ReadSignal2/1 -> ADC_5v_ID9_P29/1
  ANLG_ReadSignal3/1 -> ADC_5v_ID0_P69/1
  ANLG_ReadSignal4/1 -> ADC_5v_ID1_P59/1
  ANLG_ReadSignal5/1 -> ADC_5v_ID3_P49/1
  ANLG_ReadSignal6/1 -> ADC_5v_ID5_P50/1
  ANLG_ReadSignal7/1 -> Power_Supply24v/1
  ANLG_ReadSignal8/1 -> ADC_5v_ID6_P39/1
  ANLG_ReadSignal9/1 -> ADC_5v_ID7_P40/1
  ANLG_ReadSignal10/1 -> ADC_5v_ID12_P73/1
  ANLG_ReadSignal11/1 -> ADC_5v_ID10_P75/1
  ANLG_ReadSignal12/1 -> ADC_5v_ID11_P74/1
  ANLG_ReadSignal14/1 -> ADC_5v_ID14_P71/1
  ANLG_ReadSignal15/1 -> ADC_5v_ID15_P80/1
  ANLG_ReadSignal16/1 -> ADC_5v_ID16_P79/1
  ANLG_ReadSignal17/1 -> ADC_5v_ID17_P78/1
  ANLG_ReadSignal18/1 -> ADC_5v_ID18_P77/1
  ANLG_ReadSignal19/1 -> ADC_5v_ID19_P76/1
  ANLG_ReadSignal20/1 -> ADC_5v_ID20_P70/1
  ANLG_ReadSignal21/1 -> Temp1/1
  ANLG_ReadSignal22/1 -> Temp2/1
  IO_ReadDigitalInput/1 -> DIN_P61_AH/1
  IO_ReadDigitalInput1/1 -> DIN_P51_AH/1
  IO_ReadDigitalInput2/1 -> DIN_P22_AH/1
  IO_ReadDigitalInput3/1 -> DIN_P34_AL/1
  IO_ReadDigitalInput5/1 -> DIN_P42_AH/1
  IO_ReadDigitalInput6/1 -> DIN_P21_AH/1
  IO_ReadDigitalInput7/1 -> DIN_P31_AH/1
  IO_ReadDigitalInput17/1 -> DIN_P41_AH/1
  IO_ReadDigitalInput9/1 -> DIN_P25_AL/1
  IO_ReadDigitalInput8/1 -> DIN_P37_AH/1
  IO_ReadDigitalInput11/1 -> DIN_P35_AL/1
  IO_ReadDigitalInput10/1 -> DIN_P26_AL/1
  IO_ReadDigitalInput13/1 -> DIN_P36_AL/1
  IO_ReadDigitalInput12/1 -> DIN_P33_AH/1
  IO_ReadDigitalInput16/1 -> DIN_P28_AL/1
  IO_ReadDigitalInput14/1 -> DIN_P24_AH/1
  IO_ReadDigitalInput18/1 -> DIN_P38_AL/1
  IO_ReadDigitalInput/2 -> Terminator/1
  Ground/1 -> IO_ReadDigitalInput/2, IO_ReadDigitalInput/1
  Ground1/1 -> IO_ReadDigitalInput1/2, IO_ReadDigitalInput1/1
  Ground2/1 -> IO_ReadDigitalInput2/2, IO_ReadDigitalInput2/1
  Ground3/1 -> IO_ReadDigitalInput3/1, IO_ReadDigitalInput3/2
  Ground4/1 -> IO_ReadDigitalInput4/2, IO_ReadDigitalInput4/1
  Ground5/1 -> IO_ReadDigitalInput5/2, IO_ReadDigitalInput5/1
  Ground6/1 -> IO_ReadDigitalInput6/2, IO_ReadDigitalInput6/1
  Ground7/1 -> IO_ReadDigitalInput7/2, IO_ReadDigitalInput7/1
  Ground8/1 -> IO_ReadDigitalInput15/2, IO_ReadDigitalInput15/1
  Ground9/1 -> IO_ReadDigitalInput17/2, IO_ReadDigitalInput17/1
  Ground10/1 -> IO_ReadDigitalInput8/2, IO_ReadDigitalInput8/1
  Ground11/1 -> IO_ReadDigitalInput9/1, IO_ReadDigitalInput9/2
  IO_ReadDigitalInput2/2 -> Terminator2/1
  IO_ReadDigitalInput3/2 -> Terminator3/1
  IO_ReadDigitalInput6/2 -> Terminator6/1
  IO_ReadDigitalInput7/2 -> Terminator7/1
  IO_ReadDigitalInput15/2 -> Terminator8/1
  IO_ReadDigitalInput17/2 -> Terminator9/1
  IO_ReadDigitalInput8/2 -> Terminator10/1
  IO_ReadDigitalInput9/2 -> Terminator11/1
  IO_ReadDigitalInput11/2 -> Terminator13/1
  IO_ReadDigitalInput12/2 -> Terminator14/1
  IO_ReadDigitalInput13/2 -> Terminator15/1
  IO_ReadDigitalInput14/2 -> Terminator16/1
  IO_ReadDigitalInput16/2 -> Terminator17/1
  IO_ReadDigitalInput18/2 -> Terminator18/1
  Ground12/1 -> IO_ReadDigitalInput10/1, IO_ReadDigitalInput10/2
  Ground13/1 -> IO_ReadDigitalInput11/2, IO_ReadDigitalInput11/1
  Ground14/1 -> IO_ReadDigitalInput12/2, IO_ReadDigitalInput12/1
  Ground15/1 -> IO_ReadDigitalInput13/2, IO_ReadDigitalInput13/1
  Ground16/1 -> IO_ReadDigitalInput14/2, IO_ReadDigitalInput14/1
  Ground17/1 -> IO_ReadDigitalInput16/1, IO_ReadDigitalInput16/2
  Ground18/1 -> IO_ReadDigitalInput18/1, IO_ReadDigitalInput18/2
  Ground19/1 -> IO_ReadPwm/2, IO_ReadPwm/1
  IO_ReadPwm/1 -> PWM_IN_P13_Freq/1
  IO_ReadPwm/2 -> PWM_IN_P13_Duty/1
  ECU_HSD2_OUT2_P6/1 -> IO_WriteDigitalOutput16/1
  ECU_HSD2_OUT2_P4/1 -> IO_WriteDigitalOutput1/1
  HSDResetPin/1 -> IO_WriteDigitalOutput6/1
  P8/1 -> IO_WriteDigitalOutput9/1
  ECU_HSD2_OUT2_P2/1 -> IO_WriteDigitalOutput8/1
  ECU_HSD2_OUT2_P20/1 -> IO_WriteDigitalOutput5/1
  Reserve2/1 -> IO_WriteDigitalOutput4/1
  LSDResetPin/1 -> Terminator20/1
  Reserve/1 -> IO_WriteDigitalOutput3/1
  ECU_HSD2_OUT2_P5/1 -> IO_WriteDigitalOutput10/1
  ECU_HSD2_OUT2_P15/1 -> IO_WriteDigitalOutput14/1
  ECU_HSD2_OUT2_10/1 -> IO_WriteDigitalOutput13/1
  ECU_HSD2_OUT2_P9/1 -> IO_WriteDigitalOutput12/1
  ECU_HSD2_OUT2_P3/1 -> IO_WriteDigitalOutput11/1
  IO_ReadPwm1/2 -> PWM_IN_P14_Duty/1
  IO_ReadPwm1/1 -> PWM_IN_P14_Freq/1
  Ground20/1 -> IO_ReadPwm1/1, IO_ReadPwm1/2
  Ground21/1 -> IO_ReadPwm2/1, IO_ReadPwm2/2
  IO_ReadPwm2/2 -> PWM_IN_P62_Duty/1
  OdoReading1/1 -> Subsystem1/2(OdoReading1)
  OdoReading2/1 -> Subsystem1/5(OdoReading2)
  OdoReading3/1 -> Subsystem1/7(OdoReading3)
  Subsystem1/9(ReadData) -> ReadData/1
  Subsystem1/8(Data_Count2) -> Data_Count2/1
  Eraseee/1 -> Subsystem1/4(Eraseee)
  Speed/1 -> Subsystem1/6(Speed)
  Subsystem1/14(D1) -> D1/1
  Subsystem1/15(D2) -> D2/1
  Subsystem1/16(D3) -> D3/1
  Subsystem1/3(Updated_Data) -> COM_WriteSignal53/1, Updated_Data/1
  Subsystem1/11(A1) -> A1/1
  Subsystem1/12(A2) -> A2/1
  Subsystem1/13(A3) -> A3/1
  Subsystem1/1(RTE_Erase_Enable) -> RTE_Erase_Enable/1
  Subsystem1/2(Erase) -> Erase/1
  Subsystem1/4(RTE_Write_Enable) -> RTE_Write_Enable/1
  Subsystem1/5(Write) -> Write/1
  Subsystem1/7(DataCount) -> DataCount/1
  Ign/1 -> Subsystem1/3(Ign)
  Subsystem1/6(Readdata2) -> Readdata2/1
  Subsystem1/10(RTE_EEPROM_Value_Read) -> RTE_EEPROM_Value_Read/1
  RTE_EEPROM_Value_Write/1 -> Subsystem1/1(RTE_EEPROM_Value_Write)
  ECU_HSD2_OUT2_P1/1 -> IO_WriteDigitalOutput15/1
  H_Bridge1_Direction/1 -> IO_WriteDigitalOutput7/1
  PWM_Out_P16_Freq/1 -> IO_SetPwm5/1
  PWM_Out_P16_Duty/1 -> Terminator19/1
  PWM_Out_P7_Duty/1 -> IO_SetPwm6/2
  PWM_Out_P7_Freq/1 -> IO_SetPwm6/1
  PWM_Out_P12_Freq/1 -> IO_SetPwm1/1
  PWM_Out_P12_Duty/1 -> IO_SetPwm1/2
  PWM_Out_P11_Duty/1 -> IO_SetPwm2/2
  PWM_Out_P11_Freq/1 -> IO_SetPwm2/1
  PWM_Out_H_Freq/1 -> IO_SetPwm3/1
  PWM_Out_H_Duty/1 -> IO_SetPwm3/2
  PWM_Out_P17_Duty/1 -> IO_SetPwm4/2
  PWM_Out_P17_Freq/1 -> IO_SetPwm4/1
  IO_ReadDigitalInput15/1 -> DIN_P23_AH/1
  IO_ReadPwm2/1 -> PWM_IN_P62_Freq/1
  Chart/1(Counter) -> COM_WriteSignal52/1, COM_WriteSignal50/1, COM_WriteSignal49/1
  ANLG_ReadSignal13/1 -> ADC_5v_ID13_P72/1
  IO_ReadDigitalInput1/2 -> Terminator1/1
  IO_ReadDigitalInput4/1 -> DIN_P27_AH/1
  IO_ReadDigitalInput4/2 -> Terminator4/1
  IO_ReadDigitalInput5/2 -> Terminator5/1
  IO_ReadDigitalInput10/2 -> Terminator12/1
  Constant12/1 -> IO_SetPwm5/2
  HBridge2_Direction_Pin/1 -> HBridge2_Direction_Pin_out/1
  HBridge2/1 -> HBridge2_Out/1
  LSD1_OUT_16_P100/1 -> LSD/1(In1)
  "LSD1_OUT_15_P107 "/1 -> LSD/2(In2)
  "LSD1_OUT_14_P105 "/1 -> LSD/3(In3)
  "LSD1_OUT_13_P114 "/1 -> LSD/4(In4)
  "LSD1_OUT_12_P112 "/1 -> LSD/5(In5)
  "LSD1_OUT_11_P121 "/1 -> LSD/6(In6)
  "LSD1_OUT_10_P119 "/1 -> LSD/7(In7)
  "LSD1_OUT_9_P128 "/1 -> LSD/8(In8)
  "LSD1_OUT_8_P101 "/1 -> LSD/9(In9)
  "LSD1_OUT_7_P103 "/1 -> LSD/10(In10)
  "LSD1_OUT_6_P94 "/1 -> LSD/11(In11)
  "LSD1_OUT_5_P96 "/1 -> LSD/12(In12)
  "LSD1_OUT_4_P87 "/1 -> LSD/13(In13)
  "LSD1_OUT_3_P88 "/1 -> LSD/14(In14)
  LSD1_OUT_2_P89/1 -> LSD/15(In15)
  LSD/1(Out1) -> LSD_Data/1
  Constant/1 -> HSD/1(In1)
  Constant1/1 -> HSD/2(In2)
  Constant3/1 -> HSD/3(In3)
  Constant4/1 -> HSD/4(In4)
  Constant5/1 -> HSD/5(In5)
  Constant6/1 -> HSD/6(In6)
  Constant2/1 -> HSD/7(In7)
  Constant7/1 -> HSD/8(In8)
  Constant8/1 -> HSD/9(In9)
  Constant9/1 -> HSD/10(In10)
  Constant10/1 -> HSD/11(In11)
  Constant11/1 -> HSD/12(In12)
  ECU_HSD5_OUT4_P108/1 -> HSD/13(In13)
  "ECU_HSD5_OUT3_P123 "/1 -> HSD/14(In14)
  ECU_HSD5_OUT2_P115/1 -> HSD/15(In15)
  ECU_HSD5_OUT1_P122/1 -> HSD/16(In16)
  HSD/1(Out1) -> HSD_Data/1
  LSD1_OUT_1_P90/1 -> Terminator21/1
  Chart1/1(out) -> LSD/16(In16)

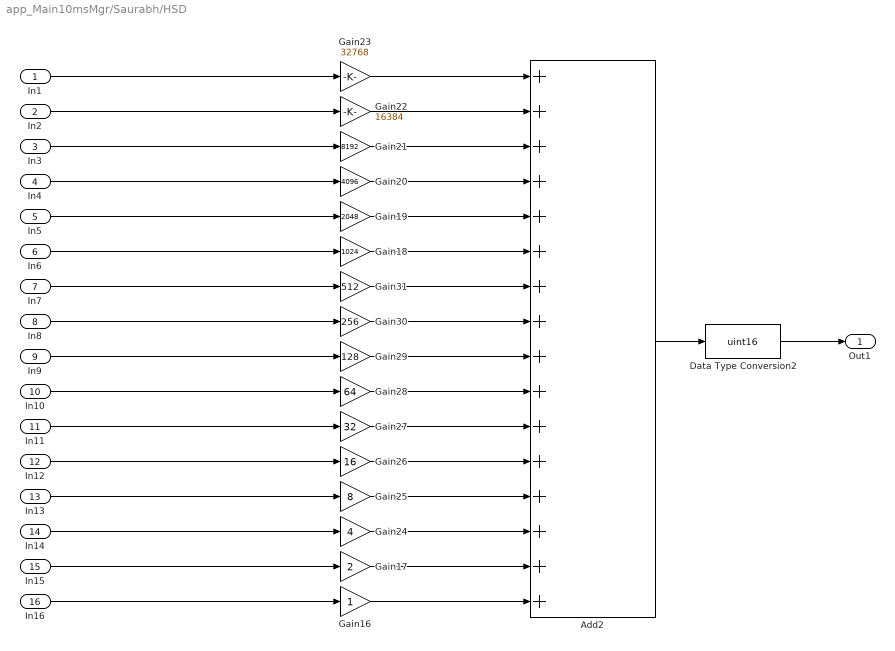
== system app_Main10msMgr/Saurabh/HSD ==
  In1 : Inport
  In2 : Inport  Port=2
  In3 : Inport  Port=3
  In4 : Inport  Port=4
  In5 : Inport  Port=5
  In6 : Inport  Port=6
  In7 : Inport  Port=7
  In8 : Inport  Port=8
  In9 : Inport  Port=9
  In10 : Inport  Port=10
  In11 : Inport  Port=11
  In12 : Inport  Port=12
  In13 : Inport  Port=13
  In14 : Inport  Port=14
  In15 : Inport  Port=15
  In16 : Inport  Port=16
  Add2 : Sum  Inputs=++++++++++++++++
  Data Type Conversion2 : DataTypeConversion  OutDataTypeStr=uint16
  Gain16 : Gain
  Gain17 : Gain  Gain=2
  Gain18 : Gain  Gain=1024
  Gain19 : Gain  Gain=2048
  Gain20 : Gain  Gain=4096
  Gain21 : Gain  Gain=8192
  Gain22 : Gain  Gain=16384
  Gain23 : Gain  Gain=32768
  Gain24 : Gain  Gain=4
  Gain25 : Gain  Gain=8
  Gain26 : Gain  Gain=16
  Gain27 : Gain  Gain=32
  Gain28 : Gain  Gain=64
  Gain29 : Gain  Gain=128
  Gain30 : Gain  Gain=256
  Gain31 : Gain  Gain=512
  Out1 : Outport
  wires:
  Gain22/1 -> Add2/2
  Add2/1 -> Data Type Conversion2/1
  Gain17/1 -> Add2/15
  Gain28/1 -> Add2/10
  Gain21/1 -> Add2/3
  Gain18/1 -> Add2/6
  In13/1 -> Gain25/1
  Gain29/1 -> Add2/9
  In15/1 -> Gain17/1
  In10/1 -> Gain28/1
  Gain23/1 -> Add2/1
  Gain30/1 -> Add2/8
  Gain16/1 -> Add2/16
  Gain24/1 -> Add2/14
  Gain20/1 -> Add2/4
  Gain19/1 -> Add2/5
  Gain27/1 -> Add2/11
  Gain31/1 -> Add2/7
  Gain25/1 -> Add2/13
  In9/1 -> Gain29/1
  In4/1 -> Gain20/1
  Gain26/1 -> Add2/12
  In8/1 -> Gain30/1
  In11/1 -> Gain27/1
  In12/1 -> Gain26/1
  Data Type Conversion2/1 -> Out1/1
  In5/1 -> Gain19/1
  In6/1 -> Gain18/1
  In2/1 -> Gain22/1
  In14/1 -> Gain24/1
  In3/1 -> Gain21/1
  In7/1 -> Gain31/1
  In16/1 -> Gain16/1
  In1/1 -> Gain23/1

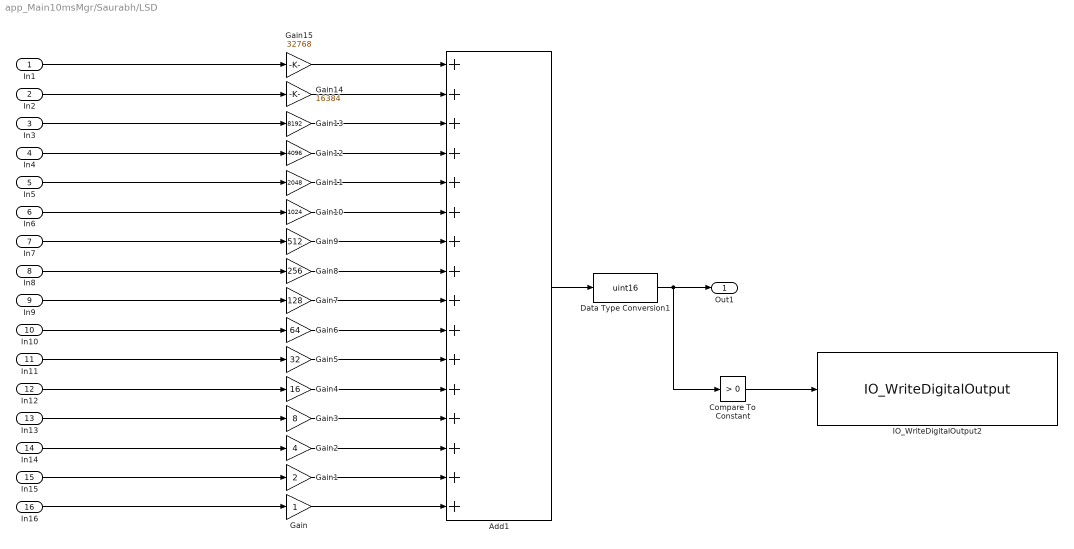
== system app_Main10msMgr/Saurabh/LSD ==
  In1 : Inport
  In2 : Inport  Port=2
  In3 : Inport  Port=3
  In4 : Inport  Port=4
  In5 : Inport  Port=5
  In6 : Inport  Port=6
  In7 : Inport  Port=7
  In8 : Inport  Port=8
  In9 : Inport  Port=9
  In10 : Inport  Port=10
  In11 : Inport  Port=11
  In12 : Inport  Port=12
  In13 : Inport  Port=13
  In14 : Inport  Port=14
  In15 : Inport  Port=15
  In16 : Inport  Port=16
  Add1 : Sum  Inputs=++++++++++++++++
  Compare To Constant : simulink/Logic and Bit Operations/Compare To Constant  relop=>  const=0  OutDataTypeStr=boolean
  Data Type Conversion1 : DataTypeConversion  OutDataTypeStr=uint16
  Gain : Gain
  Gain1 : Gain  Gain=2
  Gain10 : Gain  Gain=1024
  Gain11 : Gain  Gain=2048
  Gain12 : Gain  Gain=4096
  Gain13 : Gain  Gain=8192
  Gain14 : Gain  Gain=16384
  Gain15 : Gain  Gain=32768
  Gain2 : Gain  Gain=4
  Gain3 : Gain  Gain=8
  Gain4 : Gain  Gain=16
  Gain5 : Gain  Gain=32
  Gain6 : Gain  Gain=64
  Gain7 : Gain  Gain=128
  Gain8 : Gain  Gain=256
  Gain9 : Gain  Gain=512
  IO_WriteDigitalOutput2 : Lib_SiftProbe_deVCU_IO/IO_WriteDigitalOutput  PARAM_ID=ECU_DOUT_NONAME_PIN_LSDRESETPIN
      settings: SourceProductName=deMCD - SiftProbe_deVCU
  Out1 : Outport
  wires:
  Gain8/1 -> Add1/8
  Gain13/1 -> Add1/3
  Gain3/1 -> Add1/13
  Gain1/1 -> Add1/15
  In2/1 -> Gain14/1
  In14/1 -> Gain2/1
  Gain5/1 -> Add1/11
  Gain14/1 -> Add1/2
  Gain11/1 -> Add1/5
  Gain/1 -> Add1/16
  In10/1 -> Gain6/1
  Gain12/1 -> Add1/4
  Gain2/1 -> Add1/14
  In16/1 -> Gain/1
  Gain4/1 -> Add1/12
  Gain9/1 -> Add1/7
  In13/1 -> Gain3/1
  Gain15/1 -> Add1/1
  Gain7/1 -> Add1/9
  In4/1 -> Gain12/1
  In6/1 -> Gain10/1
  In11/1 -> Gain5/1
  Add1/1 -> Data Type Conversion1/1
  Gain6/1 -> Add1/10
  Gain10/1 -> Add1/6
  In12/1 -> Gain4/1
  In8/1 -> Gain8/1
  In9/1 -> Gain7/1
  In7/1 -> Gain9/1
  In1/1 -> Gain15/1
  In15/1 -> Gain1/1
  In3/1 -> Gain13/1
  Data Type Conversion1/1 -> Compare To Constant/1, Out1/1
  In5/1 -> Gain11/1
  Compare To Constant/1 -> IO_WriteDigitalOutput2/1

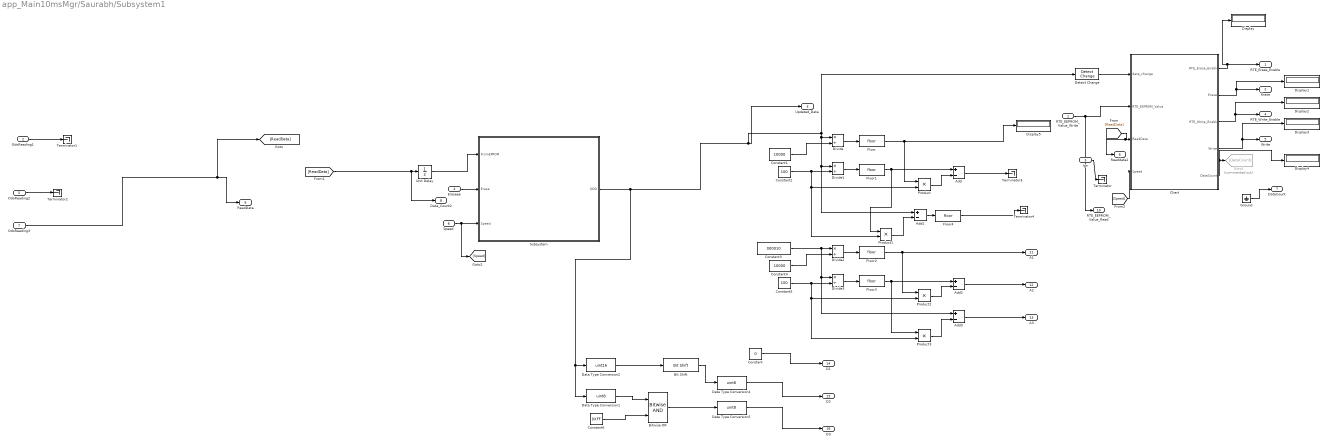
== system app_Main10msMgr/Saurabh/Subsystem1 ==
  RTE_EEPROM_Value_Write : Inport
  OdoReading1 : Inport  Port=2
  Ign : Inport  Port=3
  Eraseee : Inport  Port=4
  OdoReading2 : Inport  Port=5
  Speed : Inport  Port=6
  OdoReading3 : Inport  Port=7
  Add{,1..3} (4 alike) : Sum  Inputs=+-
  Bit Shift : hdlsllib/Logic and Bit Operations/Bit Shift  mode=Shift Right Logical  N=8
      settings: SourceProductName=Simulink
  Bitwise OR : simulink/Logic and Bit Operations/Bitwise Operator  logicop=AND  UseBitMask=off  NumInputPorts=2  BitMask=bin2dec('11011001')  BitMaskRealWorld=Stored Integer
  Chart : Stateflow chart  BlockKeywords=__PRM__SERIALIZED__DATA__:Stateflow Chart,Stateflow Diagram  TreatAsAtomicUnit=on
  Constant : Constant  Value=0
  Constant1 : Constant  Value=10000
  Constant2 : Constant  Value=100
  Constant3 : Constant  Value=000010
  Constant4 : Constant  Value=10000
  Constant5 : Constant  Value=100
  Constant6 : Constant  Value=0XFF  OutDataTypeStr=uint8
  Data Type Conversion1 : DataTypeConversion  OutDataTypeStr=uint8
  Data Type Conversion2 : DataTypeConversion  OutDataTypeStr=uint16
  Data Type Conversion4 : DataTypeConversion  OutDataTypeStr=uint8
  Data Type Conversion5 : DataTypeConversion  OutDataTypeStr=uint8
  Detect Change : simulink/Logic and Bit Operations/Detect Change  vinit=0  OutDataTypeStr=boolean
  Display{,1..5} (6 alike) : Display
  Divide{,1..3} (4 alike) : Product  Inputs=*/
  Floor{,1..4} (5 alike) : Rounding
  Goto1 : Goto  Commented=on  GotoTag=DataCount
  Ground : Ground
  Product{,1..3} (4 alike) : Product
  Subsystem : Subsystem
  Terminator{,1..4} (5 alike) : Terminator
  Unit Delay : UnitDelay  SampleTime=-1  HasFrameUpgradeWarning=on
  RTE_Erase_Enable : Outport
  Erase : Outport  Port=2
  Updated_Data : Outport  Port=3
  RTE_Write_Enable : Outport  Port=4
  Write : Outport  Port=5
  Readdata2 : Outport  Port=6
  DataCount : Outport  Port=7
  Data_Count2 : Outport  Port=8
  ReadData : Outport  Port=9
  RTE_EEPROM_Value_Read : Outport  Port=10
  A1 : Outport  Port=11
  A2 : Outport  Port=12
  A3 : Outport  Port=13
  D1 : Outport  Port=14
  D2 : Outport  Port=15
  D3 : Outport  Port=16
  wires:
  Floor1/1 -> Product1/1, Add/1
  Product3/1 -> Add3/2
  RTE_EEPROM_Value_Write/1 -> Chart/2(RTE_EEPROM_Value), RTE_EEPROM_Value_Read/1
  Divide/1 -> Floor/1
  Data Type Conversion1/1 -> Bitwise OR/1
  OdoReading2/1 -> Terminator2/1
  Constant5/1 -> Product2/2, Product3/2, Divide3/2
  Speed/1 -> [Speed], Subsystem/3(Speed)
  Bit Shift/1 -> Data Type Conversion4/1
  Constant6/1 -> Bitwise OR/2
  Data Type Conversion2/1 -> Bit Shift/1
  [ReadData] -> Readdata2/1, Chart/3(ReadData)
  Floor4/1 -> Terminator4/1
  Add/1 -> Terminator3/1
  Chart/5(DataCount) -> Display4/1, Goto1/1
  OdoReading1/1 -> Terminator1/1
  Data Type Conversion5/1 -> D3/1
  Constant/1 -> D1/1
  Data Type Conversion4/1 -> D2/1
  Divide3/1 -> Floor3/1
  Bitwise OR/1 -> Data Type Conversion5/1
  Ground/1 -> DataCount/1
  Ign/1 -> Terminator/1
  Subsystem/1(ODO) -> Data Type Conversion2/1, Data Type Conversion1/1, Updated_Data/1, Add1/1, Divide1/1, Divide/1, Detect Change/1
  Chart/3(RTE_Write_Enable) -> RTE_Write_Enable/1, Display2/1
  Constant2/1 -> Divide1/2, Product1/2, Product/2
  Constant4/1 -> Divide2/2
  [ReadData] -> Data_Count2/1, Unit Delay/1
  Floor/1 -> Display5/1, Product/1
  [Speed] -> Chart/4(Speed)
  OdoReading3/1 -> ReadData/1, [ReadData]
  Divide2/1 -> Floor2/1
  Eraseee/1 -> Subsystem/2(Erase)
  Constant1/1 -> Divide/2
  Detect Change/1 -> Chart/1(data_change)
  Chart/2(Erase) -> Erase/1, Display1/1
  Unit Delay/1 -> Subsystem/1(FromEPROM)
  Floor2/1 -> A1/1, Product2/1
  Chart/1(RTE_Erase_Enable) -> RTE_Erase_Enable/1, Display/1
  Product/1 -> Add/2
  Floor3/1 -> Add2/1, Product3/1
  Product2/1 -> Add2/2
  Product1/1 -> Add1/2
  Constant3/1 -> Divide2/1, Divide3/1, Add3/1
  Add2/1 -> A2/1
  Add1/1 -> Floor4/1
  Add3/1 -> A3/1
  Chart/4(Write) -> Write/1, Display3/1
  Divide1/1 -> Floor1/1

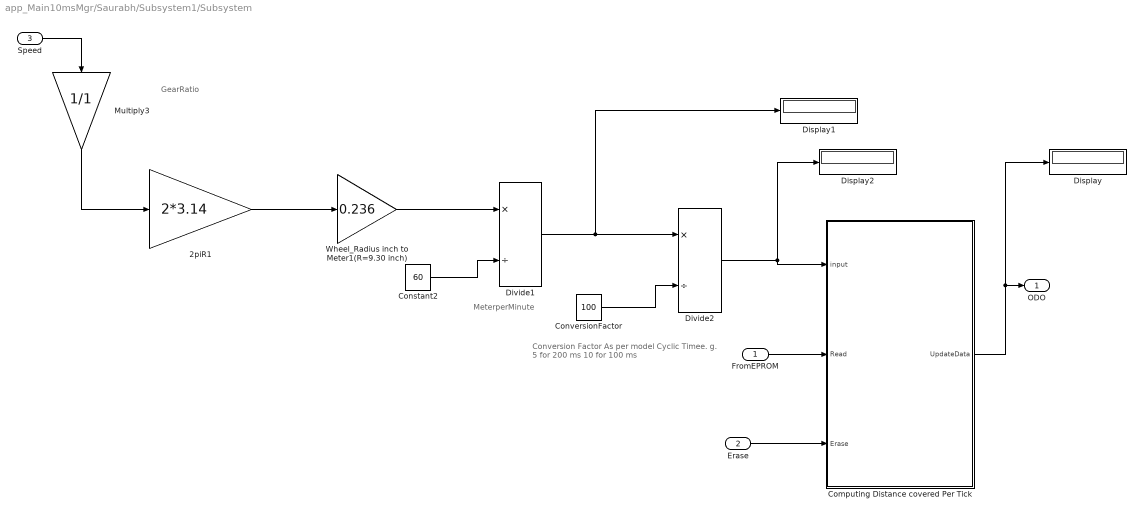
== system app_Main10msMgr/Saurabh/Subsystem1/Subsystem ==
  note: GearRatio
  note: Conversion Factor As per model Cyclic Timee.
      | g. 5 for 200 ms
      | 10 for 100 ms
  note: MeterperMinute
  FromEPROM : Inport
  Erase : Inport  Port=2
  Speed : Inport  Port=3
  2piR1 : Gain  Gain=2*3.14  OutDataTypeStr=int16  LockScale=on
  Computing Distance covered Per Tick : Stateflow chart  TreatAsAtomicUnit=on
  Constant2 : Constant  Value=60
  ConversionFactor : Constant  Value=100  OutDataTypeStr=double
  Display : Display
  Display1 : Display
  Display2 : Display
  Divide1 : Product  Inputs=*/
  Divide2 : Product  Inputs=*/
  Multiply3 : Gain  Gain=1/1
  Wheel_Radius inch to Meter1(R=9.30 inch) : Gain  Gain=0.236  OutDataTypeStr=int16  LockScale=on
  ODO : Outport
  wires:
  Divide1/1 -> Display1/1, Divide2/1
  ConversionFactor/1 -> Divide2/2
  Multiply3/1 -> 2piR1/1
  Wheel_Radius inch to Meter1(R=9.30 inch)/1 -> Divide1/1
  Constant2/1 -> Divide1/2
  2piR1/1 -> Wheel_Radius inch to Meter1(R=9.30 inch)/1
  Divide2/1 -> Display2/1, Computing Distance covered Per Tick/1(input)
  Computing Distance covered Per Tick/1(UpdateData) -> Display/1, ODO/1
  FromEPROM/1 -> Computing Distance covered Per Tick/2(Read)
  Erase/1 -> Computing Distance covered Per Tick/3(Erase)
  Speed/1 -> Multiply3/1

== stateflow chart app_Main10msMgr/Saurabh/Chart ==
  state X
    Counter=Counter+1;
  (default) -> X
  (junction 3) -> X : [Counter>=100]{Counter=0;}
  X -> (junction 3) : [after(1,sec)]
  data: Counter output =0

== stateflow chart app_Main10msMgr/Saurabh/Chart1 ==
  state OFF
    out=0;
  state ON
    out=1;
  (default) -> OFF
  ON -> OFF : [after(0.01,sec)]
  OFF -> ON : [after(0.01,sec)]
  data: out output

== stateflow chart app_Main10msMgr/Saurabh/Subsystem1/Chart ==
  state Read [commented out]
    state Read1 [commented out]
      en:
    state Read2 [commented out]
      en:
    state Read3 [commented out]
      en:
    (default) -> Read1 [commented out]
    Read1 -> Read2 [commented out]
    Read2 -> Read3 [commented out]
  state Init
    RTE_Erase_Enable = 0;
    Erase = 0;
    RTE_Write_Enable = 0;
    Write = 0;
  state ReadFormat
    en:
    DataCount=ReadData;
  state Write
    state Erase
      en:
      RTE_Erase_Enable = 1;
    state Erase1
      en:
      RTE_Erase_Enable = 0;
    state Erase2
      en:
      Erase = 1;
    state Erase3
      en:
      Erase = 0;
    state Write
      en:
      RTE_Write_Enable = 1;
    state Write1
      en:
      RTE_Write_Enable = 0;
    state Write2
      en:
      Write = 1;
    state Write3
      en:
      Write = 0;
    (default) -> Erase
    (junction 47) -> Erase
    (junction 45) -> (junction 47) : [data_change]
    Erase -> Erase1 : after(500, msec)
    Erase1 -> Erase2 : after(500, msec)
    Erase2 -> Erase3 : after(500, msec)
    Erase3 -> Write.Write : after(500, msec)
    Write.Write -> Write1 : after(500, msec)
    Write1 -> Write2 : after(500, msec)
    Write2 -> Write3 : after(500, msec)
    Write3 -> (junction 45) [order 2] : [after(500, msec)]
  state SameValue [commented out]
    en:
    RTE_Write_Enable = 0;
    RTE_Erase_Enable = 0;
  (default) -> Read [commented out]
  (default) -> Init
  Write3 -> Init [order 1] : [~Speed]
  Init -> (junction 76) : [after(500,msec)]
  (junction 76) -> ReadFormat : [Speed>0 && data_change ]
  ReadFormat -> Write : [after(500,msec)]
  Read3 -> (junction 16) [commented out]
  (junction 16) -> ? [commented out] : [RTE_EEPROM_Value ~= data_change]
  (junction 16) -> SameValue [commented out]
  data: RTE_Erase_Enable output; data_change input; RTE_EEPROM_Value input; Erase output =0; RTE_Write_Enable output =0; Write output =0; DataCount output =0; ReadData input; Speed input

== stateflow chart app_Main10msMgr/Saurabh/Subsystem1/Subsystem/Computing Distance covered Per Tick ==
  state Default
    state Default
      UpdateData=Read;
    state step1
      UpdateData=UpdateData+input;
    (default) -> Default.Default
    Default.Default -> step1 : [after(500,msec)]
    step1 -> step1
  state Erase
    UpdateData=20;
  (default) -> Default
  Erase -> Default : [~Erase]
  Default -> Erase : [Erase]
  data: input input; UpdateData output =0; Read input; Erase input
